simulink model "Train_with_data"  (R2021b)
settings: Solver=FixedStepAuto  StartTime=0.0  StopTime=2  FixedStep=1/1000  RelTol=1e-3  EnableMultiTasking=on
libraries: rllib x1
settings Model: Creator=Ammar  LastModifiedBy=vic-b
settings SolverCC: AlgebraicLoopSolver=TrustRegion  PositivePriorityOrder=on  AutoInsertRateTranBlk=on
settings OptimizationCC: EnhancedBackFolding=on  PassReuseOutputArgsThreshold=0  MaxStackSize=64  OptimizeBlockOrder=speed  DifferentSizesBufferReuse=on  OptimizationCustomize=off
settings DebuggingCC: ParameterTunabilityLossMsg=error  SFMachineParentedDataDiag=warning  ArithmeticOperatorsInVariantConditions=warning
settings HardwareCC: ProdBitPerPointer=32  ProdBitPerSizeT=32  ProdBitPerPtrDiffT=32  ProdLargestAtomicInteger=Long  ProdLargestAtomicFloat=Double  ProdWordSize=32  ProdHWDeviceType=ARM Compatible->ARM Cortex  UseEmbeddedCoderFeatures=off  UseSimulinkCoderFeatures=off
settings SFSimCC: SimUseLocalCustomCode=off  MATLABDynamicMemAlloc=off  CustomCodeUndefinedFunction=UseInterfaceOnly  SimTargetLang=C++
settings RTWCC: Description=Embedded Coder  SystemTargetFile=ert.tlc  HardwareBoard=Raspberry Pi  TLCOptions="-aInlineSetEventsForThisBaseRateFcn=TLC_FALSE -aSuppressMultiTaskScheduler=TLC_FALSE  -aRateBasedStepFcn=0"  TemplateMakefile=ert_default_tmf  GenerateReport=on  RTWUseLocalCustomCode=off  Toolchain=GNU GCC Embedded Linux  BuildConfiguration=Faster Runs  LaunchReport=on
settings CodeAppCC: ForceParamTrailComments=on  OperatorAnnotations=on
settings ERTTargetCC: ERTCustomFileBanners=off  SupportContinuousTime=on  SupportNonInlinedSFcns=on  RemoveResetFunc=off  SupportVariableSizeSignals=on  ModelStepFunctionPrototypeControlCompliant=off

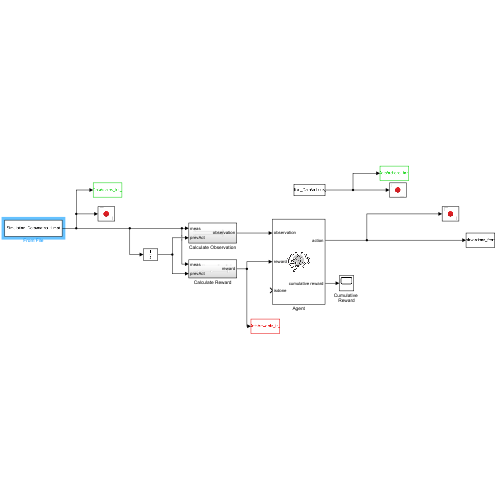
[thumbnail: Simulink's stored preview of the top-level diagram]
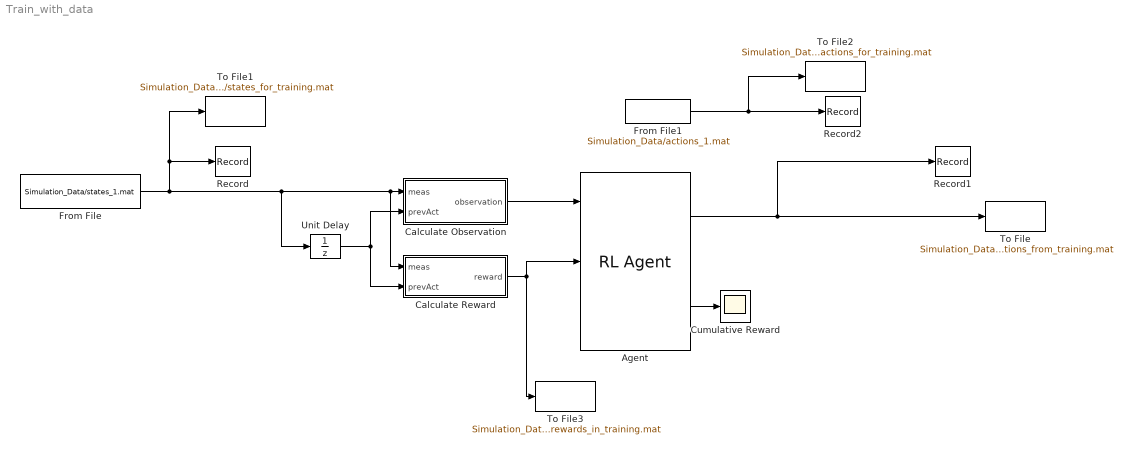
== system Train_with_data ==
  Agent : rllib/RL Agent  Agent=agent  ExternalActionAsInput=off  ProvideCumRwd=on  TreatAsDirectFeedthrough=on
      settings: SourceProductName=Reinforcement Learning
  Calculate Observation : Subsystem
  Calculate Reward : Subsystem
  Cumulative Reward : Scope
  From File : FromFile  FileName=Simulation_Data/states_1.mat  SampleTime=0.004
  From File1 : FromFile  FileName=Simulation_Data/actions_1.mat  SampleTime=0
  Record : Record  FileSettingsInternal="{\"entries\":[{\"content\":{\"excelSettings\":{\"content\":{},\"type\":\"Streamout.ExcelSettings\"}},\"type\":\"Streamout.FileSettingStorage\",\"uuid\":\"936d60d6-7a7a-4cd1-aea4-65dcbf71db82\"}],\"packageUris\":[\"http://schema.mathworks.com/mf0/streamout_blocks/R2020a\"],\"version\":\"1.0\"}"  SignalsInternal="{\"entries\":[{\"content\":{\"signals\":[{\"content\":{\"blockPath\":[\"Train_with_data/Record\"],\"channel\":[],\"dimensions\":[1,1],\"domain\":\"Train_with_data/Record\",\"lineColor\":\"#22b573\",\"plots\":[1],\"port\":1,\"sid\":[],\"signalID\":19,\"signalName\":\"From File\"},\"type\":\"RecordBlkView.Signal\",\"uuid\":\"85532b55-e050-4d8b-a013-679f798d5f89\"}]},\"type\":\"RecordBlkView.InputSignals\",\"uuid\":\"b8413d51-9687-4c1b-896d-4e5ddde64e2a\"}],\"packageUris\":[\"http://schema.mathworks.com/mf0/streamout_blocks/R2020a\"],\"version\":\"1.0\"}"  VisualizationBindings="{\"sparklinesplugin\":{\"info\":[{\"bindingParametersList\":[],\"subplotID\":1}]}}"
  Record1 : Record  FileSettingsInternal="{\"entries\":[{\"content\":{\"excelSettings\":{\"content\":{},\"type\":\"Streamout.ExcelSettings\"}},\"type\":\"Streamout.FileSettingStorage\",\"uuid\":\"78dea6c4-5f7f-4c36-90f9-bb1f87949c7e\"}],\"packageUris\":[\"http://schema.mathworks.com/mf0/streamout_blocks/R2020a\"],\"version\":\"1.0\"}"  SignalsInternal="{\"entries\":[{\"content\":{\"signals\":[{\"content\":{\"blockPath\":[\"Train_with_data/Record1\"],\"channel\":[],\"dimensions\":[1,1],\"domain\":\"Train_with_data/Record1\",\"lineColor\":\"#0072bd\",\"plots\":[1],\"port\":1,\"sid\":[],\"signalID\":14,\"signalName\":\"Agent:1\"},\"type\":\"RecordBlkView.Signal\",\"uuid\":\"a945bbb3-122c-433e-831f-718719ed1cdf\"}]},\"type\":\"RecordBlkView.InputSignals\",\"uuid\":\"bbec69a5-8b88-4624-bf50-e65cbbae0fbc\"}],\"packageUris\":[\"http://schema.mathworks.com/mf0/streamout_blocks/R2020a\"],\"version\":\"1.0\"}"  VisualizationBindings="{\"sparklinesplugin\":{\"info\":[{\"bindingParametersList\":[],\"subplotID\":1}]}}"
  Record2 : Record  FileSettingsInternal="{\"entries\":[{\"content\":{\"excelSettings\":{\"content\":{},\"type\":\"Streamout.ExcelSettings\"}},\"type\":\"Streamout.FileSettingStorage\",\"uuid\":\"a38788ef-e5bf-49cf-abb1-ec645aa90a5b\"}],\"packageUris\":[\"http://schema.mathworks.com/mf0/streamout_blocks/R2020a\"],\"version\":\"1.0\"}"  SignalsInternal="{\"entries\":[{\"content\":{\"signals\":[{\"content\":{\"blockPath\":[\"Train_with_data/Record2\"],\"channel\":[],\"dimensions\":[1,1],\"domain\":\"Train_with_data/Record2\",\"lineColor\":\"#d95319\",\"plots\":[1],\"port\":1,\"sid\":[],\"signalID\":9,\"signalName\":\"From File1\"},\"type\":\"RecordBlkView.Signal\",\"uuid\":\"6b3edf29-d9c6-4857-8a69-fedd9b0c68bf\"}]},\"type\":\"RecordBlkView.InputSignals\",\"uuid\":\"c0c74674-af02-4de0-823e-583efab9172d\"}],\"packageUris\":[\"http://schema.mathworks.com/mf0/streamout_blocks/R2020a\"],\"version\":\"1.0\"}"  VisualizationBindings="{\"sparklinesplugin\":{\"info\":[{\"bindingParametersList\":[],\"subplotID\":1}]}}"
  To File : ToFile  Filename=Simulation_Data/actions_from_training.mat  SaveFormat=Timeseries
  To File1 : ToFile  Filename=Simulation_Data/states_for_training.mat  SaveFormat=Timeseries
  To File2 : ToFile  Filename=Simulation_Data/actions_for_training.mat  SaveFormat=Timeseries
  To File3 : ToFile  Filename=Simulation_Data/rewards_in_training.mat  SaveFormat=Timeseries
  Unit Delay : UnitDelay  SampleTime=-1  HasFrameUpgradeWarning=on
  wires:
  From File/1 -> Unit Delay/1, Calculate Reward/1(meas), Calculate Observation/1(meas), Record/1, To File1/1
  Calculate Observation/1(observation) -> Agent/1
  Unit Delay/1 -> Calculate Observation/2(prevAct), Calculate Reward/2(prevAct)
  Agent/2 -> Cumulative Reward/1
  Agent/1 -> To File/1, Record1/1
  Calculate Reward/1(reward) -> Agent/2, To File3/1
  From File1/1 -> To File2/1, Record2/1

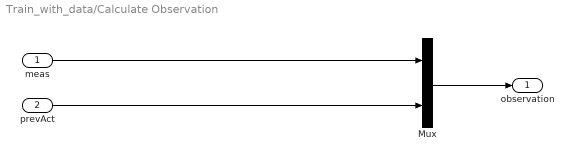
== system Train_with_data/Calculate Observation ==
  meas : Inport
  prevAct : Inport  Port=2
  Mux : Mux  Inputs=2
  observation : Outport  VectorParamsAs1DForOutWhenUnconnected=off
  wires:
  Mux/1 -> observation/1
  meas/1 -> Mux/1
  prevAct/1 -> Mux/2

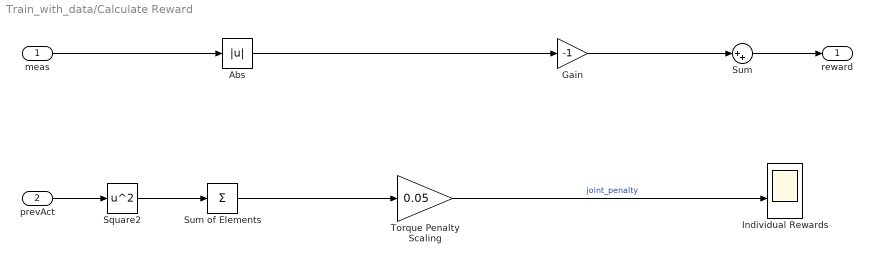
== system Train_with_data/Calculate Reward ==
  meas : Inport
  prevAct : Inport  Port=2
  Abs : Abs
  Gain : Gain  Gain=-1
  Individual Rewards : Scope  NumInputPorts=4
  Square2 : Math  Operator=square  SignedPower=on  SaturateOnIntegerOverflow=on
  Sum : Sum  Inputs=|++
  Sum of Elements : Sum  Inputs=+
  Torque Penalty Scaling : Gain  Gain=0.05
  reward : Outport  VectorParamsAs1DForOutWhenUnconnected=off
  wires:
  meas/1 -> Abs/1
  Sum of Elements/1 -> Torque Penalty Scaling/1
  prevAct/1 -> Square2/1
  Square2/1 -> Sum of Elements/1
  Torque Penalty Scaling/1 -> Individual Rewards/3  "joint_penalty"
  Abs/1 -> Gain/1
  Gain/1 -> Sum/1
  Sum/1 -> reward/1
